simulink model "lab6"  (R2016a)
settings: Solver=VariableStepAuto  StartTime=0.0  StopTime=10.0  RelTol=1e-3
settings Model: Creator=Student  LastModifiedBy=Student

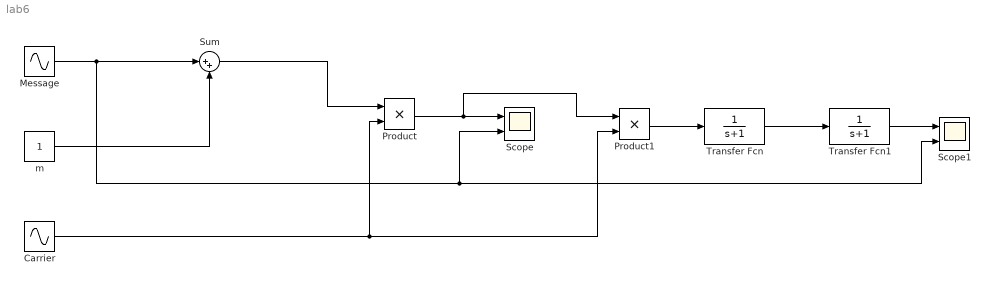
== system lab6 ==
  Carrier : Sin  Frequency=2*pi*25  SampleTime=1/5000
  Message : Sin  Frequency=2*pi  SampleTime=1/5000  Offset=1/5000
  Product : Product
  Product1 : Product
  Scope : Scope  NumInputPorts=2
  Scope1 : Scope  NumInputPorts=2
  Sum : Sum  Inputs=|++
  Transfer Fcn : TransferFcn  Denominator=[1 1]
  Transfer Fcn1 : TransferFcn  Denominator=[1 1]
  m : Constant
  wires:
  Sum/1 -> Product/1
  Message/1 -> Sum/1, Scope1/2, Scope/2
  m/1 -> Sum/2
  Carrier/1 -> Product1/2, Product/2
  Product/1 -> Product1/1, Scope/1
  Product1/1 -> Transfer Fcn/1
  Transfer Fcn/1 -> Transfer Fcn1/1
  Transfer Fcn1/1 -> Scope1/1
